simulink model "Experiment_4_1_PRBS"  (R2018a)
settings: Solver=FixedStepAuto  StartTime=0.0  StopTime=50  FixedStep=Ts  RelTol=1e-8  AbsTol=1e-8  EnableMultiTasking=on
undefined symbols (not defined in the file or in its folder): Ts
libraries: EEE481Arduino x5
settings Model: SimulationMode=external  ExtModeTrigDuration=2  Creator=vaggarw7  LastModifiedBy=abhig
settings SolverCC: AutoScaleAbsTol=off
settings OptimizationCC: PassReuseOutputArgsAs=Individual arguments  MaxStackSize=64
settings DebuggingCC: ParameterTunabilityLossMsg=error
settings HardwareCC: ProdBitPerPointer=32  ProdBitPerSizeT=32  ProdBitPerPtrDiffT=32  ProdLargestAtomicInteger=Long  ProdLargestAtomicFloat=Double  ProdWordSize=32  ProdHWDeviceType=ARM Compatible->ARM Cortex
settings SFSimCC: MATLABDynamicMemAlloc=off
settings RTWCC: SystemTargetFile=ert.tlc  HardwareBoard=Arduino Due  TLCOptions=-aInlineSetEventsForThisBaseRateFcn=TLC_FALSE -aSuppressMultiTaskScheduler=TLC_FALSE -aRateBasedStepFcn=1  TemplateMakefile=ert_default_tmf  GenerateReport=on  Toolchain=Arduino ARM  BuildConfiguration=Faster Runs  IncludeHyperlinkInReport=on  LaunchReport=on  GenerateTraceInfo=on  GenerateTraceReport=on  GenerateTraceReportSl=on  GenerateTraceReportSf=on  GenerateTraceReportEml=on
settings CodeAppCC: ForceParamTrailComments=on  IgnoreCustomStorageClasses=off  OperatorAnnotations=on  SimulinkDataObjDesc=on  SFDataObjDesc=on  MATLABFcnDesc=on  InsertBlockDesc=on  StateflowObjectComments=on  MATLABSourceComments=on
settings ERTTargetCC: SupportContinuousTime=on  SupportVariableSizeSignals=on

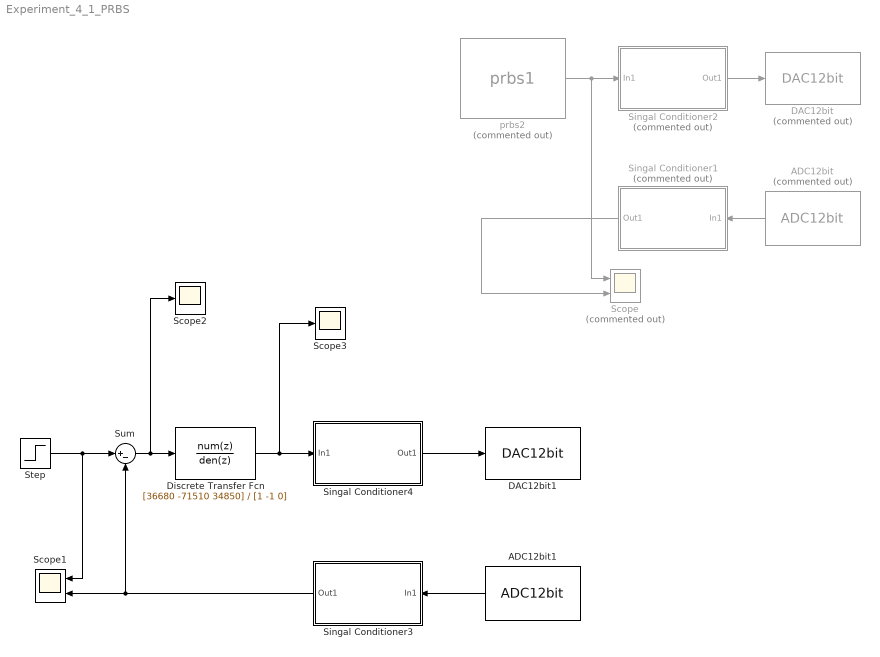
== system Experiment_4_1_PRBS ==
  ADC12bit : EEE481Arduino/ADC12bit  Commented=on  pinNum=0  Tsa=Ts
      settings: SourceProductName=EEE 481 Arduino
  ADC12bit1 : EEE481Arduino/ADC12bit  pinNum=0  Tsa=Ts
      settings: SourceProductName=EEE 481 Arduino
  DAC12bit : EEE481Arduino/DAC12bit  Commented=on  Tsa=Ts  DACNum=0
      settings: SourceProductName=EEE 481 Arduino
  DAC12bit1 : EEE481Arduino/DAC12bit  Tsa=Ts  DACNum=0
      settings: SourceProductName=EEE 481 Arduino
  Discrete Transfer Fcn : DiscreteTransferFcn  Numerator=[36680 -71510 34850]  Denominator=[1 -1 0]
  Scope : Scope  Commented=on  NumInputPorts=2
  Scope1 : Scope  NumInputPorts=2
  Scope2 : Scope
  Scope3 : Scope
  Singal Conditioner1 : Subsystem  Commented=on  mask{out_min=-pi/2, out_max=pi/2, in_min=0.56, in_max=2.76}
      mask prompts: out_min "Minimum Value of Output Signal"; out_max "Maximum Value of Output Signal"; in_min "Minimum Value of Input Signal"; in_max "Maximum Value of Input Signal"
  Singal Conditioner2 : Subsystem  Commented=on  mask{out_min=0.56, out_max=2.76, in_min=-255, in_max=255}
      mask prompts: out_min "Minimum Value of Output Signal"; out_max "Maximum Value of Output Signal"; in_min "Minimum Value of Input Signal"; in_max "Maximum Value of Input Signal"
  Singal Conditioner3 : Subsystem  mask{out_min=-pi/2, out_max=pi/2, in_min=0.56, in_max=2.76}
      mask prompts: out_min "Minimum Value of Output Signal"; out_max "Maximum Value of Output Signal"; in_min "Minimum Value of Input Signal"; in_max "Maximum Value of Input Signal"
  Singal Conditioner4 : Subsystem  mask{out_min=0.56, out_max=2.76, in_min=-255, in_max=255}
      mask prompts: out_min "Minimum Value of Output Signal"; out_max "Maximum Value of Output Signal"; in_min "Minimum Value of Input Signal"; in_max "Maximum Value of Input Signal"
  Step : Step  Time=25  After=pi/6  SampleTime=Ts
  Sum : Sum  Inputs=|+-
  prbs2 : EEE481Arduino/prbs1  Commented=on  Tsa=Ts  Tsw=Tsw  Lz=18  Lv=255  Nc=1  initLevel=0
      settings: SourceProductName=EEE 481 Arduino
  wires:
  ADC12bit/1 -> Singal Conditioner1/1(In1)
  prbs2/1 -> Scope/1, Singal Conditioner2/1(In1)
  Singal Conditioner2/1(Out1) -> DAC12bit/1
  Singal Conditioner1/1(Out1) -> Scope/2
  Step/1 -> Sum/1, Scope1/1
  Singal Conditioner3/1(Out1) -> Sum/2, Scope1/2
  Sum/1 -> Scope2/1, Discrete Transfer Fcn/1
  Discrete Transfer Fcn/1 -> Scope3/1, Singal Conditioner4/1(In1)
  ADC12bit1/1 -> Singal Conditioner3/1(In1)
  Singal Conditioner4/1(Out1) -> DAC12bit1/1

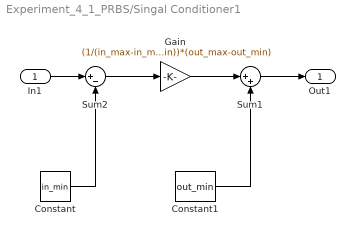
== system Experiment_4_1_PRBS/Singal Conditioner1 ==
  In1 : Inport
  Constant : Constant  Value=in_min
  Constant1 : Constant  Value=out_min
  Gain : Gain  Gain=(1/(in_max-in_min))*(out_max-out_min)
  Sum1 : Sum  Inputs=|++
  Sum2 : Sum  Inputs=|+-
  Out1 : Outport
  wires:
  Sum2/1 -> Gain/1
  In1/1 -> Sum2/1
  Constant1/1 -> Sum1/2
  Sum1/1 -> Out1/1
  Gain/1 -> Sum1/1
  Constant/1 -> Sum2/2

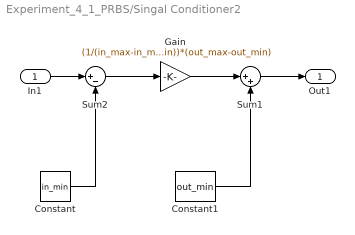
== system Experiment_4_1_PRBS/Singal Conditioner2 ==
  In1 : Inport
  Constant : Constant  Value=in_min
  Constant1 : Constant  Value=out_min
  Gain : Gain  Gain=(1/(in_max-in_min))*(out_max-out_min)
  Sum1 : Sum  Inputs=|++
  Sum2 : Sum  Inputs=|+-
  Out1 : Outport
  wires:
  Constant/1 -> Sum2/2
  Gain/1 -> Sum1/1
  Sum1/1 -> Out1/1
  Constant1/1 -> Sum1/2
  In1/1 -> Sum2/1
  Sum2/1 -> Gain/1

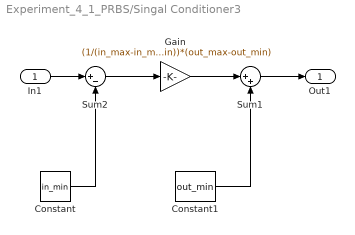
== system Experiment_4_1_PRBS/Singal Conditioner3 ==
  In1 : Inport
  Constant : Constant  Value=in_min
  Constant1 : Constant  Value=out_min
  Gain : Gain  Gain=(1/(in_max-in_min))*(out_max-out_min)
  Sum1 : Sum  Inputs=|++
  Sum2 : Sum  Inputs=|+-
  Out1 : Outport
  wires:
  Sum2/1 -> Gain/1
  In1/1 -> Sum2/1
  Constant1/1 -> Sum1/2
  Sum1/1 -> Out1/1
  Gain/1 -> Sum1/1
  Constant/1 -> Sum2/2

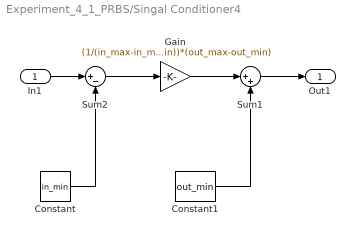
== system Experiment_4_1_PRBS/Singal Conditioner4 ==
  In1 : Inport
  Constant : Constant  Value=in_min
  Constant1 : Constant  Value=out_min
  Gain : Gain  Gain=(1/(in_max-in_min))*(out_max-out_min)
  Sum1 : Sum  Inputs=|++
  Sum2 : Sum  Inputs=|+-
  Out1 : Outport
  wires:
  Constant/1 -> Sum2/2
  Gain/1 -> Sum1/1
  Sum1/1 -> Out1/1
  Constant1/1 -> Sum1/2
  In1/1 -> Sum2/1
  Sum2/1 -> Gain/1
